simulink model "Panics1"  (R2014a)
settings: Solver=ode3  StartTime=0.0  StopTime=10.0  RelTol=1e-3
undefined symbols (not defined in the file or in its folder): Engine, Trans
libraries: simulink x2
settings Model: Creator=swami  LastModifiedBy=swami

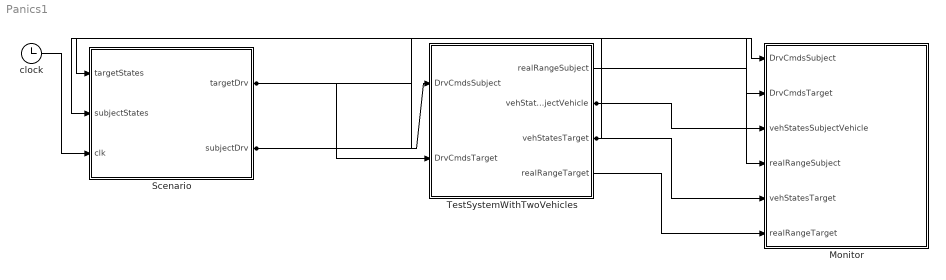
== system Panics1 ==
  Monitor : Subsystem
  Scenario : Stateflow chart  TreatAsAtomicUnit=on
  TestSystemWithTwoVehicles : Subsystem
  clock : Clock
  wires:
  Scenario/1(targetDrv) -> TestSystemWithTwoVehicles/2(DrvCmdsTarget), Monitor/2(DrvCmdsTarget)
  Scenario/2(subjectDrv) -> TestSystemWithTwoVehicles/1(DrvCmdsSubject), Monitor/1(DrvCmdsSubject)
  TestSystemWithTwoVehicles/3(vehStatesTarget) -> Scenario/1(targetStates), Monitor/5(vehStatesTarget)
  TestSystemWithTwoVehicles/2(vehStatesSubjectVehicle) -> Scenario/2(subjectStates), Monitor/3(vehStatesSubjectVehicle)
  clock/1 -> Scenario/3(clk)
  TestSystemWithTwoVehicles/1(realRangeSubject) -> Monitor/4(realRangeSubject)
  TestSystemWithTwoVehicles/4(realRangeTarget) -> Monitor/6(realRangeTarget)

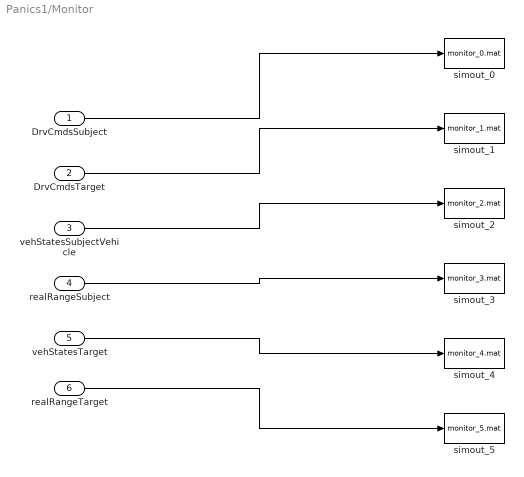
== system Panics1/Monitor ==
  DrvCmdsSubject : Inport
  DrvCmdsTarget : Inport  Port=2
  vehStatesSubjectVehicle : Inport  Port=3
  realRangeSubject : Inport  Port=4
  vehStatesTarget : Inport  Port=5
  realRangeTarget : Inport  Port=6
  simout_0 : ToFile  Filename=monitor_0.mat  MatrixName=DrvCmdsSubject  SaveFormat=Timeseries
  simout_1 : ToFile  Filename=monitor_1.mat  MatrixName=DrvCmdsTarget  SaveFormat=Timeseries
  simout_2 : ToFile  Filename=monitor_2.mat  MatrixName=vehStatesSubjectVehicle  SaveFormat=Timeseries
  simout_3 : ToFile  Filename=monitor_3.mat  MatrixName=realRangeSubject  SaveFormat=Timeseries
  simout_4 : ToFile  Filename=monitor_4.mat  MatrixName=vehStatesTarget  SaveFormat=Timeseries
  simout_5 : ToFile  Filename=monitor_5.mat  MatrixName=realRangeTarget  SaveFormat=Timeseries
  wires:
  DrvCmdsSubject/1 -> simout_0/1
  DrvCmdsTarget/1 -> simout_1/1
  vehStatesSubjectVehicle/1 -> simout_2/1
  realRangeSubject/1 -> simout_3/1
  vehStatesTarget/1 -> simout_4/1
  realRangeTarget/1 -> simout_5/1

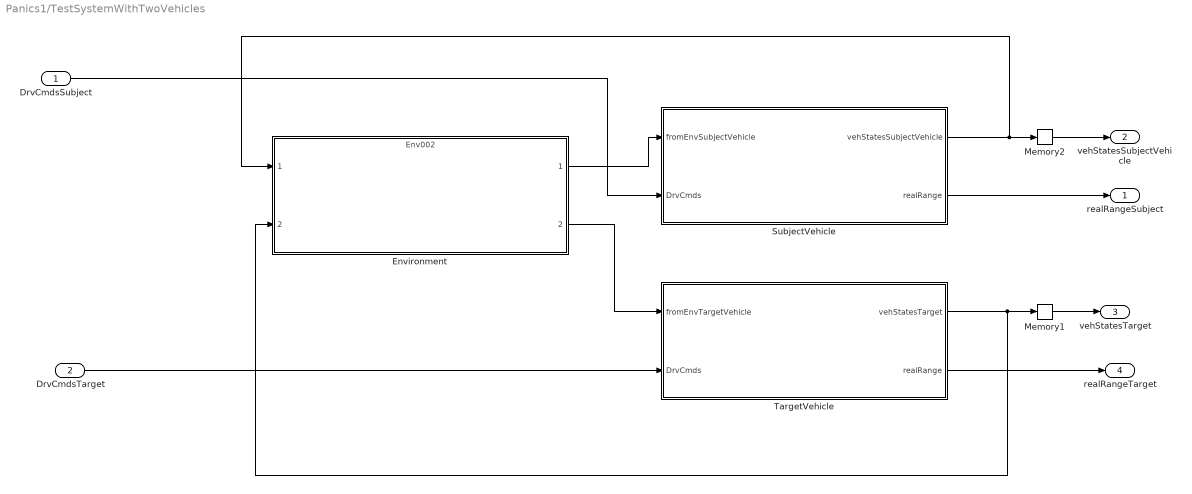
== system Panics1/TestSystemWithTwoVehicles ==
  DrvCmdsSubject : Inport  OutDataTypeStr=double
  DrvCmdsTarget : Inport  Port=2
  Environment : ModelReference  ModelNameDialog=Env002  SimulationMode=Normal  Variant=on  OverrideUsingVariant=ECR1_varEnv002  ModelReferenceVersion=1.10  CopyOfModelName=Env002  DefaultDataLogging=on
      settings: AttributesFormatString=%<ActiveVariant>
  Memory1 : Memory
  Memory2 : Memory
  SubjectVehicle : Subsystem
  TargetVehicle : Subsystem
  realRangeSubject : Outport
  vehStatesSubjectVehicle : Outport  Port=2
  vehStatesTarget : Outport  Port=3
  realRangeTarget : Outport  Port=4
  wires:
  Memory1/1 -> vehStatesTarget/1
  Memory2/1 -> vehStatesSubjectVehicle/1
  DrvCmdsSubject/1 -> SubjectVehicle/2(DrvCmds)
  DrvCmdsTarget/1 -> TargetVehicle/2(DrvCmds)
  TargetVehicle/2(realRange) -> realRangeTarget/1
  SubjectVehicle/2(realRange) -> realRangeSubject/1
  SubjectVehicle/1(vehStatesSubjectVehicle) -> Memory2/1, Environment/1
  Environment/1 -> SubjectVehicle/1(fromEnvSubjectVehicle)
  Environment/2 -> TargetVehicle/1(fromEnvTargetVehicle)
  TargetVehicle/1(vehStatesTarget) -> Memory1/1, Environment/2

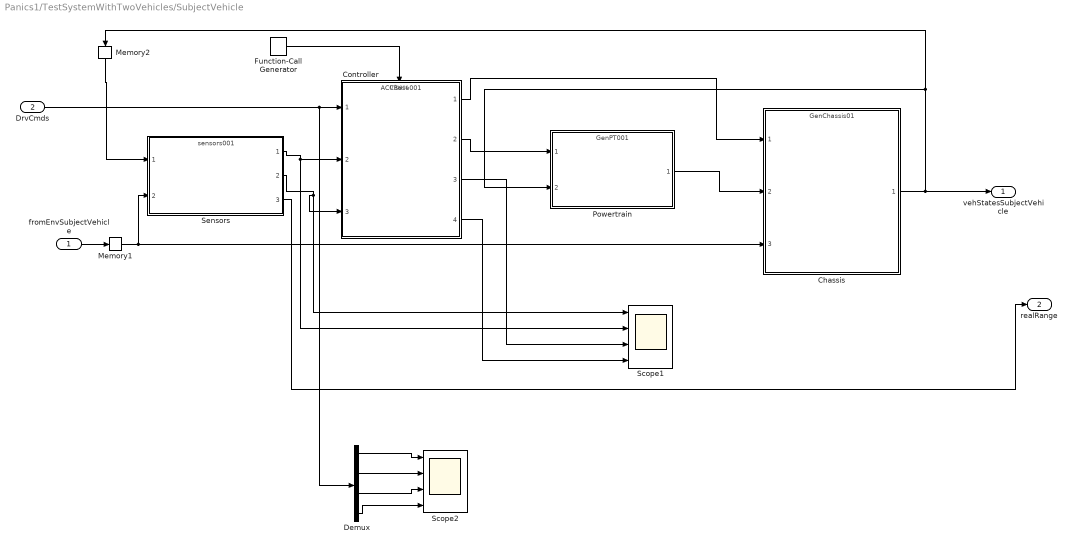
== system Panics1/TestSystemWithTwoVehicles/SubjectVehicle ==
  fromEnvSubjectVehicle : Inport
  DrvCmds : Inport  Port=2
  Chassis : ModelReference  ModelNameDialog=GenChassis01  ParameterArgumentNames=Chassis  ParameterArgumentValues=ChassisSubject  SimulationMode=Normal  Variant=on  OverrideUsingVariant=ECR1_varChassis01  ModelReferenceVersion=1.19  CopyOfModelName=GenChassis01  DefaultDataLogging=on
      settings: AttributesFormatString=%<ActiveVariant>
  Controller : ModelReference  ModelNameDialog=ACCBase001  ParameterArgumentNames=pACC  ParameterArgumentValues=pACCBase  SimulationMode=Normal  Variant=on  OverrideUsingVariant=ECR1_varACCBase001  ModelReferenceVersion=1.92  CopyOfModelName=ACCBase001  DefaultDataLogging=on  TriggerPortName=Trigger  TriggerPortTriggerType=function-call  TriggerPortStatesWhenEnabling=held
      settings: AttributesFormatString=%<ActiveVariant>
  Demux : Demux
  Function-Call Generator : simulink/Ports & Subsystems/Function-Call Generator  sample_time=0.1  numberOfIterations=1
  Memory1 : Memory
  Memory2 : Memory
  Powertrain : ModelReference  ModelNameDialog=GenPT001  ParameterArgumentNames=Trans,Engine  ParameterArgumentValues=Trans,Engine  SimulationMode=Normal  Variant=on  OverrideUsingVariant=ECR1_varGenPT001  ModelReferenceVersion=1.23  CopyOfModelName=GenPT001  DefaultDataLogging=on
      settings: AttributesFormatString=%<ActiveVariant>
  Scope1 : Scope  NumInputPorts=4
  Scope2 : Scope  NumInputPorts=4
  Sensors : ModelReference  ModelNameDialog=sensors001  SimulationMode=Normal  Variant=on  OverrideUsingVariant=ECR1_varSensor001  ModelReferenceVersion=1.21  CopyOfModelName=sensors001  DefaultDataLogging=on
      settings: AttributesFormatString=%<ActiveVariant>
  vehStatesSubjectVehicle : Outport
  realRange : Outport  Port=2
  wires:
  Demux/4 -> Scope2/4
  Demux/1 -> Scope2/1
  Demux/3 -> Scope2/3
  Demux/2 -> Scope2/2
  Sensors/3 -> realRange/1
  Controller/4 -> Scope1/4
  Controller/3 -> Scope1/3
  Function-Call Generator/1 -> Controller/Trigger
  Memory1/1 -> Chassis/3, Sensors/2
  fromEnvSubjectVehicle/1 -> Memory1/1
  Memory2/1 -> Sensors/1
  DrvCmds/1 -> Controller/1, Demux/1
  Sensors/2 -> Scope1/1, Controller/3
  Sensors/1 -> Controller/2, Scope1/2
  Controller/1 -> Chassis/1
  Powertrain/1 -> Chassis/2
  Controller/2 -> Powertrain/1
  Chassis/1 -> vehStatesSubjectVehicle/1, Memory2/1, Powertrain/2

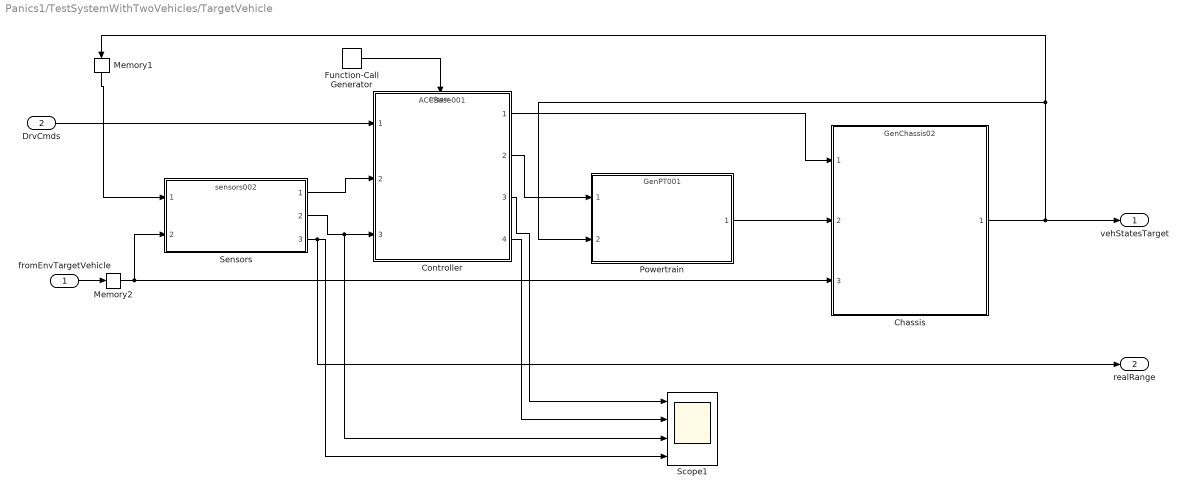
== system Panics1/TestSystemWithTwoVehicles/TargetVehicle ==
  fromEnvTargetVehicle : Inport
  DrvCmds : Inport  Port=2
  Chassis : ModelReference  ModelNameDialog=GenChassis02  ParameterArgumentNames=Chassis  ParameterArgumentValues=ChassisTarget  SimulationMode=Normal  Variant=on  OverrideUsingVariant=ECR1_varChassis02  ModelReferenceVersion=1.19  CopyOfModelName=GenChassis02  DefaultDataLogging=on
      settings: AttributesFormatString=%<ActiveVariant>
  Controller : ModelReference  ModelNameDialog=ACCBase001  ParameterArgumentNames=pACC  ParameterArgumentValues=pACCBase  SimulationMode=Normal  Variant=on  OverrideUsingVariant=ECR1_var0005  ModelReferenceVersion=1.92  CopyOfModelName=ACCBase001  DefaultDataLogging=on  TriggerPortName=Trigger  TriggerPortTriggerType=function-call  TriggerPortStatesWhenEnabling=held
      settings: AttributesFormatString=%<ActiveVariant>
  Function-Call Generator : simulink/Ports & Subsystems/Function-Call Generator  sample_time=0.1  numberOfIterations=1
  Memory1 : Memory
  Memory2 : Memory
  Powertrain : ModelReference  ModelNameDialog=GenPT001  ParameterArgumentNames=Trans,Engine  ParameterArgumentValues=Trans,Engine  SimulationMode=Normal  Variant=on  OverrideUsingVariant=ECR1_varGenPT001  ModelReferenceVersion=1.23  CopyOfModelName=GenPT001  DefaultDataLogging=on
      settings: AttributesFormatString=%<ActiveVariant>
  Scope1 : Scope  NumInputPorts=4
  Sensors : ModelReference  ModelNameDialog=sensors002  SimulationMode=Normal  Variant=on  OverrideUsingVariant=varObject1  ModelReferenceVersion=1.19  CopyOfModelName=sensors002  DefaultDataLogging=on
      settings: AttributesFormatString=%<ActiveVariant>
  vehStatesTarget : Outport
  realRange : Outport  Port=2
  wires:
  Sensors/3 -> Scope1/4, realRange/1
  Controller/4 -> Scope1/2
  Controller/3 -> Scope1/1
  Function-Call Generator/1 -> Controller/Trigger
  Memory2/1 -> Chassis/3, Sensors/2
  Memory1/1 -> Sensors/1
  Chassis/1 -> Powertrain/2, Memory1/1, vehStatesTarget/1
  fromEnvTargetVehicle/1 -> Memory2/1
  Controller/2 -> Powertrain/1
  Powertrain/1 -> Chassis/2
  Controller/1 -> Chassis/1
  DrvCmds/1 -> Controller/1
  Sensors/1 -> Controller/2
  Sensors/2 -> Controller/3, Scope1/3

== stateflow chart Panics1/Scenario ==
  state Act_TargetVehicle [parallel]
    settings: executionOrder=1
    state Act_TargetVehicle_Step1
    state Act_TargetVehicle_Step2
      state Act_TargetVehicle_Step2_1
        entry: targetDrv = [0,1,0,0];
        state Act_TargetVehicle_Step2_1_1
        state Act_TargetVehicle_Step2_1_2
          state Act_TargetVehicle_Step2_1_2_1
            entry: targetDrv = [0,1,0,0];
            entry: Act_TargetVehicle_Step2_1_2_1_stpClk = clk;
          state Act_TargetVehicle_Step2_1_2_2
            entry: targetDrv = [0,0,0,0];
          (default) -> Act_TargetVehicle_Step2_1_2_1
          Act_TargetVehicle_Step2_1_2_1 -> Act_TargetVehicle_Step2_1_2_2 : [clk - Act_TargetVehicle_Step2_1_2_1_stpClk >= 2]
        (default) -> Act_TargetVehicle_Step2_1_1
        Act_TargetVehicle_Step2_1_1 -> Act_TargetVehicle_Step2_1_2 : [targetStates(1) - subjectStates(1) < 50]
      state Act_TargetVehicle_Step2_2
        entry: targetDrv = [0,0,1,50];
      (default) -> Act_TargetVehicle_Step2_1
      Act_TargetVehicle_Step2_1 -> Act_TargetVehicle_Step2_2 : [targetStates(2) >= 50]
    (default) -> Act_TargetVehicle_Step1
    Act_TargetVehicle_Step1 -> Act_TargetVehicle_Step2 : [clk > 0]
  state Act_SubjectVehicle [parallel]
    settings: executionOrder=2
    state Act_SubjectVehicle_Step1
    state Act_SubjectVehicle_Step2
      state Act_SubjectVehicle_Step2_1
        entry: subjectDrv = [0,1,0,0];
      state Act_SubjectVehicle_Step2_2
        entry: subjectDrv = [0,0,1,60];
      (default) -> Act_SubjectVehicle_Step2_1
      Act_SubjectVehicle_Step2_1 -> Act_SubjectVehicle_Step2_2 : [subjectStates(2) >= 60]
    (default) -> Act_SubjectVehicle_Step1
    Act_SubjectVehicle_Step1 -> Act_SubjectVehicle_Step2 : [clk > 0]
  data: targetStates input; subjectStates input; clk input; targetDrv output; subjectDrv output; Act_TargetVehicle_Step2_1_2_1_stpClk local
